simulink model "ML_UAV_3D_2"  (R2018a)
settings: Solver=ode4  StartTime=0.0  StopTime=130  FixedStep=Ts  MaxStep=2*T  MinStep=T  RelTol=1e-4
values from neighbouring files (symbols this model uses):
  Ac = 0.0331    [init_ML_UAV_3D_2.m]
  Am1_LPF = sysd.denominator{1}    [init_ML_UAV_3D_2.m]
  Am2_LPF = sysd.denominator{1}    [init_ML_UAV_3D_2.m]
  Am_coup_LPF = sysd.denominator{1}    [init_ML_UAV_3D_2.m]
  Amp_sf = 3    [init_ML_UAV_3D_2.m]
  Amp_sf_rp = 0.05*uav.m*g    [init_ML_UAV_3D_2.m]
  Bm1_LPF = sysd.numerator{1}    [init_ML_UAV_3D_2.m]
  Bm2_LPF = sysd.numerator{1}    [init_ML_UAV_3D_2.m]
  Bm_coup_LPF = sysd.numerator{1}    [init_ML_UAV_3D_2.m]
  C_S = [5;5;9]*10^-3    [init_ML_UAV_3D_2.m]
  Cd_u = 0.2    [init_ML_UAV_3D_2.m]
  dc_M_p = 6.7    [init_ML_UAV_3D_2.m]
  eps_V = 0.5    [init_ML_UAV_3D_2.m]
  g = 9.81    [init_ML_UAV_3D_2.m]
  gamma_d_p = (2*0.3/0.03*2*0.2*12/4)/10    (= 2.4)    [init_ML_UAV_3D_2.m]
  k3 = 24    [init_ML_UAV_3D_2.m]
  k4 = 0.8    [init_ML_UAV_3D_2.m]
  min_sf = 5    [init_ML_UAV_3D_2.m]
  min_sf_rp = 0.35*uav.m*g    [init_ML_UAV_3D_2.m]
  OMEGA_FILTER_OUTER = 40    [estimation.m]
  T_init = 10    [init_ML_UAV_3D_2.m]
  Tc = 1/500    (= 0.002)    [estimation.m]
  Tg = 1/ 20    (= 0.05)    [estimation.m]
  Tn = 1/500    (= 0.002)    [estimation.m]
  Ts = 1/500    (= 0.002)    [estimation.m]    (also in init_ML_UAV_3D_2.m)
  Tsc = 1/100    (= 0.01)    [estimation.m]
  Tz = 1/500    (= 0.002)    [estimation.m]
  X_GPS_offset = [0.01 0.005]    [estimation.m]
undefined symbols (not defined in the file or in its folder): Am_HPF, Am_LPF, Am_LPF2, an1, an1_v, an2, an3, Bm_HPF, Bm_LPF, Bm_LPF2, bn1, bn1_v, bn2, bn3, buoy, cable, controller, current, D_b, DiscIntNeverNeededParam, F, filters, J_u, K, kd_t, kp_t, L, Light, magnitude, MIL, Phi0, Psi0, R_b, T, Theta0, theta_q_ini, tolerences, torque_corr, uav, Vol_b, water, wave, X0_u
libraries: simulink x48, simulink_extras x10, UAV_Control x4, dspmtrx3 x2, aerolibwind2 x2
(part 3 of 6)

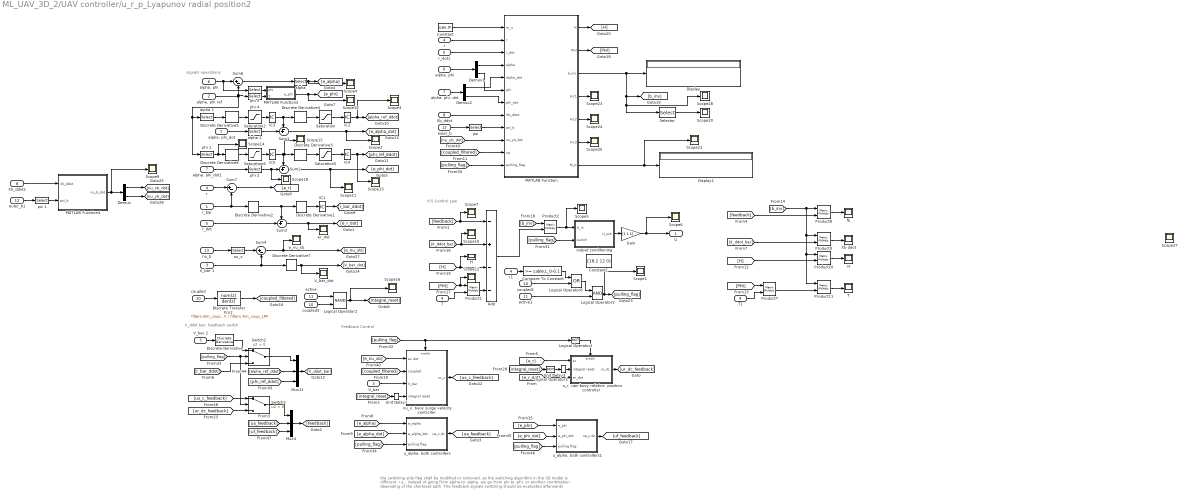
== system ML_UAV_3D_2/UAV controller/u_r_p_Lyapunov radial position2 ==
  note: the switching side flag shall be modified or removed, as the switching algorithm in the 3D model is different.
      | i.e., instead of going from alpha to -alpha, we go from phi to -phi, or another combination depending of the shorteset path.
      |
      | The feedback signals switching should be evaluated afterwards
  note: Feedback Control
  note: ICS Control Law
  note: X_ddot bar, feedbach switch
  note: signals operations
  "r_bar " : Inport
  "alpha, phi ref" : Inport  Port=2
  "V_bar " : Inport  Port=3
  r : Inport  Port=4
  r_dot : Inport  Port=5
  "alpha, phi" : Inport  Port=6
  "alpha, phi, dot" : Inport  Port=7
  Xb_ddot : Inport  Port=8
  T : Inport  Port=9
  coupled : Inport  Port=10
  active : Inport  Port=11
  euler_b : Inport  Port=12
  nu_b : Inport  Port=13
  " H " : Scope
  " H  " : Scope
  " T  " : Scope
  " alpha " : Selector  InputPortWidth=2  IndexOptions=Index vector (dialog)  Indices=1  OutputSizes=1
  " alpha 1" : Selector  InputPortWidth=2  IndexOptions=Index vector (dialog)  Indices=1  OutputSizes=1
  " alpha 2" : Selector  InputPortWidth=2  IndexOptions=Index vector (dialog)  Indices=1  OutputSizes=1
  " fb " : Scope
   phi {1..2,4..5} (4 alike) : Selector  InputPortWidth=2  IndexOptions=Index vector (dialog)  Indices=2  OutputSizes=1
  Add : Sum  Inputs=-+--
  Compare To Constant : simulink/Logic and Bit Operations/Compare To Constant  relop=>=  const=cable.L_0-0.1  OutDataTypeStr=boolean
  Constant : Constant  Value=uav.m
  Constant1 : Constant  Value=[18.2 12 0]
  Demux : Demux  Outputs=2
  Demux1 : Demux  Outputs=2
  Demux2 : Demux  Outputs=2
  Discrete Transfer Fcn2 : DiscreteTransferFcn  Numerator=filters.Bm_coup_LPF  Denominator=filters.Am_coup_LPF
  Discrete Derivative : simulink/Discrete/Discrete Derivative  gainval=1.0  ICPrevScaledInput=0.0  OutMin=[]  OutMax=[]  OutDataType=fixdt(1, 16)  OutScaling=2^-10  DoSatur=off
  Discrete Derivative1 : simulink/Discrete/Discrete Derivative  gainval=1.0  ICPrevScaledInput=uav.r_0/Ts  OutMin=[]  OutMax=[]  OutDataType=fixdt(1, 16)  OutScaling=2^-10  DoSatur=off
  Discrete Derivative2 : simulink/Discrete/Discrete Derivative  gainval=1.0  ICPrevScaledInput=uav.r_0/Ts  OutMin=[]  OutMax=[]  OutDataType=fixdt(1, 16)  OutScaling=2^-10  DoSatur=off
  Discrete Derivative3 : simulink/Discrete/Discrete Derivative  gainval=1.0  ICPrevScaledInput=alpha_bar  OutMin=[]  OutMax=[]  OutDataType=fixdt(1, 16)  OutScaling=2^-10  DoSatur=off
  Discrete Derivative4 : simulink/Discrete/Discrete Derivative  gainval=1.0  ICPrevScaledInput=alpha_bar  OutMin=[]  OutMax=[]  OutDataType=fixdt(1, 16)  OutScaling=2^-10  DoSatur=off
  Discrete Derivative5 : simulink/Discrete/Discrete Derivative  gainval=1.0  ICPrevScaledInput=uav.alpha_bar_0/Ts  OutMin=[]  OutMax=[]  OutDataType=fixdt(1, 16)  OutScaling=2^-10  DoSatur=off
  Discrete Derivative6 : simulink/Discrete/Discrete Derivative  gainval=1.0  ICPrevScaledInput=uav.phi_0/Ts  OutMin=[]  OutMax=[]  OutDataType=fixdt(1, 16)  OutScaling=2^-10  DoSatur=off
  Discrete Derivative7 : simulink/Discrete/Discrete Derivative  gainval=1.0  ICPrevScaledInput=uav.r_0/Ts  OutMin=[]  OutMax=[]  OutDataType=fixdt(1, 16)  OutScaling=2^-10  DoSatur=off
  Display : Display
  Display1 : Display
  Gain : Gain  Gain=[1 1 1]
  IC{1..5} (5 alike) : InitialCondition  Value=0
  Logical Operator1 : Logic  Operator=NOT  AllPortsSameDT=off  OutDataTypeStr=boolean
  Logical Operator2 : Logic  Operator=NAND  AllPortsSameDT=off  OutDataTypeStr=boolean
  Logical Operator3 : Logic  Operator=NOT  AllPortsSameDT=off  OutDataTypeStr=boolean
  Logical Operator5 : Logic  AllPortsSameDT=off  OutDataTypeStr=boolean
  Logical Operator6 : Logic  Operator=OR  AllPortsSameDT=off  OutDataTypeStr=boolean
  MATLAB Function : MATLAB Function  TreatAsAtomicUnit=on
  MATLAB Function2 : MATLAB Function  TreatAsAtomicUnit=on
  MATLAB Function4 : MATLAB Function  TreatAsAtomicUnit=on
  Mux11 : Mux  Inputs=3
  Mux4 : Mux  Inputs=3
  Product{1..2,7..11} (7 alike) : Product  Inputs=**  Multiplication=Matrix(*)
  Saturation : Saturate  UpperLimit=2  LowerLimit=-2
  Saturation2 : Saturate  UpperLimit=1  LowerLimit=-1
  Saturation5 : Saturate  UpperLimit=2  LowerLimit=-2
  Saturation6 : Saturate  UpperLimit=1  LowerLimit=-1
  Scope{1..7,9..16,18..21,23..25,27..28} (24 alike) : Scope
  Selector : Selector  NumberOfDimensions=2  InputPortWidth=3  IndexOptions=Index vector (dialog),Index vector (dialog)  Indices=[2 3],[3 3]  OutputSizes=1,1
  Sum1 : Sum  Inputs=-+|
  Sum2 : Sum  Inputs=-+|
  Sum3 : Sum  Inputs=-+|
  Sum4 : Sum  Inputs=|+-
  Sum6 : Sum  Inputs=|+-
  Sum7 : Sum  Inputs=|+-
  Switch2 : Switch  Criteria=u2 > Threshold
  Switch3 : Switch  Criteria=u2 > Threshold
  T1 : InportShadow  Port=9
  Unit Delay1 : UnitDelay  SampleTime=-1
  Unit Delay3 : UnitDelay  SampleTime=-1
  V_bar 1 : InportShadow  Port=3
  V_bar 2 : InportShadow  Port=3
  V_bar_dot : Scope
  "Xb ddot " : Scope
  Xb_ddot1 : InportShadow  Port=8
  active1 : InportShadow  Port=11
  "alpha, phi " : InportShadow  Port=6
  "alpha, phi_dot" : InportShadow  Port=7
  "alpha, phi_dot1" : InportShadow  Port=7
  coupled1 : InportShadow  Port=10
  coupled3 : InportShadow  Port=10
  e_nu_xb : Scope
  er_dot : Scope
  euler_b1 : InportShadow  Port=12
  nu_x : Selector  InputPortWidth=2  IndexOptions=Index vector (dialog)  Indices=1  OutputSizes=1
  "nu_x, buoy surge velocity controller" : Subsystem
  output conditioning : Subsystem
  "psi " : Selector  InputPortWidth=3  IndexOptions=Index vector (dialog)  Indices=3  OutputSizes=1
  psi 1 : Selector  InputPortWidth=3  IndexOptions=Index vector (dialog)  Indices=3  OutputSizes=1
  "r  " : InportShadow  Port=4
  r1 : InportShadow  Port=4
  r_dot1 : InportShadow  Port=5
  "u_alpha, both controllers" : Subsystem
  "u_alpha, both controllers1" : Subsystem
  "u_r, uav-buoy relative  position controller" : Subsystem
  U : Outport
  wires:
  r_dot/1 -> Sum3/2
  [feedback] -> Add/1, Scope7/1
  r_dot1/1 -> MATLAB Function/3(r_dot)
  Discrete Derivative2/1 -> Discrete Derivative1/1, Sum3/1
  Discrete Derivative4/1 -> Saturation/1
  Saturation2/1 -> IC3/1
  " alpha 1"/1 -> Discrete Derivative5/1
  Discrete Derivative5/1 -> Saturation2/1
  IC3/1 -> Discrete Derivative4/1, Sum1/1
  Saturation/1 -> IC2/1
  [coupled_filtered] -> MATLAB Function/11(cp)
  coupled3/1 -> Logical Operator2/2
  coupled/1 -> Discrete Transfer Fcn2/1
  active/1 -> Logical Operator2/1
  "alpha, phi "/1 -> " phi 5"/1, Sum6/1
  "alpha, phi ref"/1 -> " phi 1"/1, " alpha 1"/1, " phi 4"/1, Sum6/2
  Sum6/1 -> " alpha "/1
  " alpha "/1 -> Scope4/1, [e_alpha]
  MATLAB Function2/1(e_phi) -> Scope19/1, [e_phi]
  "r  "/1 -> Sum7/1
  "r_bar "/1 -> Discrete Derivative2/1, Sum7/2
  Sum7/1 -> [e_r]
  Discrete Derivative1/1 -> IC1/1
  IC2/1 -> Scope3/1, [alpha_ref_ddot]
  " phi 1"/1 -> Scope14/1, Discrete Derivative6/1
  Discrete Derivative3/1 -> Saturation5/1
  Discrete Derivative6/1 -> Saturation6/1
  IC4/1 -> Scope13/1, [phi_ref_ddot]
  Saturation6/1 -> IC5/1
  Saturation5/1 -> IC4/1
  IC1/1 -> [r_bar_ddot]
  Sum3/1 -> er_dot/1, [e_r_dot]
  "alpha, phi_dot"/1 -> " alpha 2"/1
  Sum1/1 -> Scope2/1, [e_alpha_dot]
  " alpha 2"/1 -> Sum1/2
  "alpha, phi_dot1"/1 -> " phi 2"/1
  " phi 2"/1 -> Scope18/1, Sum2/2
  IC5/1 -> Scope15/1, Discrete Derivative3/1, Sum2/1
  Sum2/1 -> [e_phi_dot], Scope11/1
  Discrete Transfer Fcn2/1 -> [coupled_filtered]
  "alpha, phi"/1 -> Demux1/1
  Demux1/1 -> MATLAB Function/4(alpha)
  Demux1/2 -> MATLAB Function/6(phi)
  Demux2/1 -> MATLAB Function/5(alpha_dot)
  Demux2/2 -> MATLAB Function/7(phi_dot)
  "alpha, phi, dot"/1 -> Demux2/1
  Xb_ddot/1 -> MATLAB Function/8(Xb_ddot)
  [pulling_flag] -> MATLAB Function/12(pulling_flag)
  r/1 -> MATLAB Function/2(r)
  [phi_ref_ddot] -> Mux11/3
  [alpha_ref_ddot] -> Mux11/2
  [pulling_flag] -> Switch2/2, Switch3/2
  Discrete Derivative/1 -> Switch2/1
  [r_bar_ddot] -> Switch2/3
  Switch2/1 -> Mux11/1
  [X_ddot_bar] -> Add/2, Scope10/1
  MATLAB Function/2(PHI) -> [PHI]
  [PHI] -> Scope12/1, Product1/1
  T/1 -> Product1/2
  Product1/1 -> Add/4
  [b_inv] -> Product2/1
  MATLAB Function/1(H) -> [H]
  Constant/1 -> MATLAB Function/1(m_u)
  [ur_dc_feedback] -> Switch3/3
  [ua_feedback] -> Mux4/2
  Logical Operator2/1 -> Scope16/1, [integral_reset]
  [e_nu_xb] -> "nu_x, buoy surge velocity controller"/1(ex dot)
  [coupled_filtered] -> "nu_x, buoy surge velocity controller"/2(coupled)
  "V_bar "/1 -> "nu_x, buoy surge velocity controller"/3(V_bar)
  [integral_reset] -> Unit Delay1/1
  "nu_x, buoy surge velocity controller"/1(ux_c) -> [ux_c_feedback]
  [e_r] -> "u_r, uav-buoy relative  position controller"/1(er)
  [integral_reset] -> Logical Operator3/1
  [e_r_dot] -> "u_r, uav-buoy relative  position controller"/3(er_dot)
  "u_r, uav-buoy relative  position controller"/1(ur_dc) -> [ur_dc_feedback]
  Logical Operator3/1 -> Unit Delay3/1
  [e_alpha] -> "u_alpha, both controllers"/1(e_alpha)
  [e_alpha_dot] -> "u_alpha, both controllers"/2(e_alpha_dot)
  "u_alpha, both controllers"/1(ua_c,dc) -> [ua_feedback]
  [ux_c_feedback] -> Switch3/1
  Switch3/1 -> Mux4/1
  [pulling_flag] -> output conditioning/2(switch)
  Unit Delay1/1 -> "nu_x, buoy surge velocity controller"/4(integral reset)
  Unit Delay3/1 -> "u_r, uav-buoy relative  position controller"/2(integral reset)
  Logical Operator1/1 -> "u_r, uav-buoy relative  position controller"/Enable
  r1/1 -> Compare To Constant/1
  active1/1 -> Logical Operator5/2
  Logical Operator6/1 -> Logical Operator5/1
  coupled1/1 -> Logical Operator6/2
  Compare To Constant/1 -> Logical Operator6/1
  Logical Operator5/1 -> Scope1/1, [pulling_flag]
  output conditioning/1(U_out) -> Gain/1
  Gain/1 -> Scope6/1, U/1
  Add/1 -> Product2/2
  [pulling_flag] -> "u_alpha, both controllers"/3(pulling flag)
  Selector/1 -> Scope20/1
  MATLAB Function/4(Hc1) -> Scope23/1
  MATLAB Function/5(Hc2) -> Scope24/1
  MATLAB Function/6(Hc3) -> Scope25/1
  MATLAB Function/3(b_inv) -> Display/1, [b_inv], Selector/1, Scope28/1
  " phi 4"/1 -> MATLAB Function2/2(phi_cmd)
  " phi 5"/1 -> MATLAB Function2/1(phi)
  [H] -> Add/3, " H  "/1
  Product2/1 -> output conditioning/1(U_in), Scope5/1
  euler_b/1 -> "psi "/1
  "psi "/1 -> MATLAB Function/9(psi_b)
  Sum4/1 -> e_nu_xb/1, [e_nu_xb]
  nu_b/1 -> nu_x/1
  [nu_yb_dot] -> MATLAB Function/10(nu_yb_dot)
  V_bar 2/1 -> Discrete Derivative/1
  [pulling_flag] -> "u_alpha, both controllers1"/3(pulling flag)
  [e_phi_dot] -> "u_alpha, both controllers1"/2(e_phi_dot)
  [e_phi] -> "u_alpha, both controllers1"/1(e_phi)
  "u_alpha, both controllers1"/1(ua_c,dc) -> [uf_feedback]
  [uf_feedback] -> Mux4/3
  Xb_ddot1/1 -> MATLAB Function4/1(Xb_ddot)
  euler_b1/1 -> psi 1/1
  psi 1/1 -> MATLAB Function4/2(psi_b)
  MATLAB Function4/1(nu_b_dot) -> Scope9/1, Demux/1
  Demux/1 -> [nu_xb_dot]
  Demux/2 -> [nu_yb_dot]
  MATLAB Function/7(M_p) -> Display1/1, Scope21/1
  [pulling_flag] -> "nu_x, buoy surge velocity controller"/Enable, Logical Operator1/1
  Mux11/1 -> [X_ddot_bar]
  Mux4/1 -> [feedback]
  [PHI] -> Product7/1
  T1/1 -> Product7/2
  Product8/1 -> " fb "/1
  [feedback] -> Product8/2
  Product7/1 -> Product11/2
  [H] -> Product10/2
  [X_ddot_bar] -> Product9/2
  [b_inv] -> Product11/1, Product10/1, Product9/1, Product8/1
  Product9/1 -> "Xb ddot "/1
  Product10/1 -> " H "/1
  Product11/1 -> " T  "/1
  nu_x/1 -> Sum4/1
  V_bar 1/1 -> Discrete Derivative7/1, Sum4/2
  Discrete Derivative7/1 -> V_bar_dot/1, [V_bar_dot]

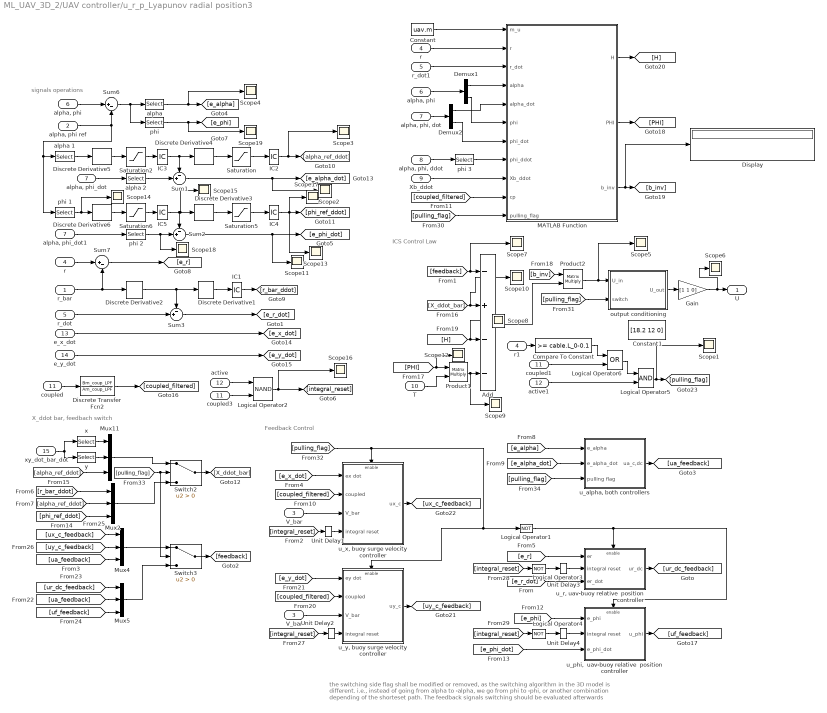
== system ML_UAV_3D_2/UAV controller/u_r_p_Lyapunov radial position3 ==
  note: the switching side flag shall be modified or removed, as the switching algorithm in the 3D model is different.
      | i.e., instead of going from alpha to -alpha, we go from phi to -phi, or another combination depending of the shorteset path.
      |
      | The feedback signals switching should be evaluated afterwards
  note: Feedback Control
  note: ICS Control Law
  note: X_ddot bar, feedbach switch
  note: signals operations
  "r_bar " : Inport
  "alpha, phi ref" : Inport  Port=2
  "V_bar " : Inport  Port=3
  r : Inport  Port=4
  r_dot : Inport  Port=5
  "alpha, phi" : Inport  Port=6
  "alpha, phi, dot" : Inport  Port=7
  "alpha, phi, ddot" : Inport  Port=8
  Xb_ddot : Inport  Port=9
  T : Inport  Port=10
  coupled : Inport  Port=11
  active : Inport  Port=12
  e_x_dot : Inport  Port=13
  e_y_dot : Inport  Port=14
  xy_dot_bar_dot : Inport  Port=15
  " alpha " : Selector  InputPortWidth=2  IndexOptions=Index vector (dialog)  Indices=1  OutputSizes=1
  " alpha 1" : Selector  InputPortWidth=2  IndexOptions=Index vector (dialog)  Indices=1  OutputSizes=1
  " alpha 2" : Selector  InputPortWidth=2  IndexOptions=Index vector (dialog)  Indices=1  OutputSizes=1
   phi {,1..3} (4 alike) : Selector  InputPortWidth=2  IndexOptions=Index vector (dialog)  Indices=2  OutputSizes=1
  " x " : Selector  InputPortWidth=2  IndexOptions=Index vector (dialog)  Indices=1  OutputSizes=1
  " y " : Selector  InputPortWidth=2  IndexOptions=Index vector (dialog)  Indices=2  OutputSizes=1
  Add : Sum  Inputs=-+--
  Compare To Constant : simulink/Logic and Bit Operations/Compare To Constant  relop=>=  const=cable.L_0-0.1  OutDataTypeStr=boolean
  Constant : Constant  Value=uav.m
  Constant1 : Constant  Value=[18.2 12 0]
  Demux1 : Demux  Outputs=2
  Demux2 : Demux  Outputs=2
  Discrete Transfer Fcn2 : DiscreteTransferFcn  Numerator=Bm_coup_LPF  Denominator=Am_coup_LPF
  Discrete Derivative1 : simulink/Discrete/Discrete Derivative  gainval=1.0  ICPrevScaledInput=uav.r_0/Ts  OutMin=[]  OutMax=[]  OutDataType=fixdt(1, 16)  OutScaling=2^-10  DoSatur=off
  Discrete Derivative2 : simulink/Discrete/Discrete Derivative  gainval=1.0  ICPrevScaledInput=uav.r_0/Ts  OutMin=[]  OutMax=[]  OutDataType=fixdt(1, 16)  OutScaling=2^-10  DoSatur=off
  Discrete Derivative3 : simulink/Discrete/Discrete Derivative  gainval=1.0  ICPrevScaledInput=alpha_bar  OutMin=[]  OutMax=[]  OutDataType=fixdt(1, 16)  OutScaling=2^-10  DoSatur=off
  Discrete Derivative4 : simulink/Discrete/Discrete Derivative  gainval=1.0  ICPrevScaledInput=alpha_bar  OutMin=[]  OutMax=[]  OutDataType=fixdt(1, 16)  OutScaling=2^-10  DoSatur=off
  Discrete Derivative5 : simulink/Discrete/Discrete Derivative  gainval=1.0  ICPrevScaledInput=uav.alpha_bar_0/Ts  OutMin=[]  OutMax=[]  OutDataType=fixdt(1, 16)  OutScaling=2^-10  DoSatur=off
  Discrete Derivative6 : simulink/Discrete/Discrete Derivative  gainval=1.0  ICPrevScaledInput=uav.phi_0/Ts  OutMin=[]  OutMax=[]  OutDataType=fixdt(1, 16)  OutScaling=2^-10  DoSatur=off
  Display : Display
  Gain : Gain  Gain=[1 1 0]
  IC{1..5} (5 alike) : InitialCondition  Value=0
  Logical Operator1 : Logic  Operator=NOT  AllPortsSameDT=off  OutDataTypeStr=boolean
  Logical Operator2 : Logic  Operator=NAND  AllPortsSameDT=off  OutDataTypeStr=boolean
  Logical Operator3 : Logic  Operator=NOT  AllPortsSameDT=off  OutDataTypeStr=boolean
  Logical Operator4 : Logic  Operator=NOT  AllPortsSameDT=off  OutDataTypeStr=boolean
  Logical Operator5 : Logic  AllPortsSameDT=off  OutDataTypeStr=boolean
  Logical Operator6 : Logic  Operator=OR  AllPortsSameDT=off  OutDataTypeStr=boolean
  MATLAB Function : MATLAB Function  TreatAsAtomicUnit=on
  Mux{2,4..5,11} (4 alike) : Mux  Inputs=3
  Product1 : Product  Inputs=**  Multiplication=Matrix(*)
  Product2 : Product  Inputs=**  Multiplication=Matrix(*)
  Saturation : Saturate  UpperLimit=2  LowerLimit=-2
  Saturation2 : Saturate  UpperLimit=1  LowerLimit=-1
  Saturation5 : Saturate  UpperLimit=2  LowerLimit=-2
  Saturation6 : Saturate  UpperLimit=1  LowerLimit=-1
  Scope{1..19} (19 alike) : Scope
  Sum1 : Sum  Inputs=-+|
  Sum2 : Sum  Inputs=-+|
  Sum3 : Sum  Inputs=-+|
  Sum6 : Sum  Inputs=|+-
  Sum7 : Sum  Inputs=|+-
  Switch2 : Switch  Criteria=u2 > Threshold
  Switch3 : Switch  Criteria=u2 > Threshold
  Unit Delay{1..4} (4 alike) : UnitDelay  SampleTime=-1
  V_bar : InportShadow  Port=3
  active1 : InportShadow  Port=12
  "alpha, phi " : InportShadow  Port=6
  "alpha, phi_dot" : InportShadow  Port=7
  "alpha, phi_dot1" : InportShadow  Port=7
  coupled1 : InportShadow  Port=11
  coupled3 : InportShadow  Port=11
  output conditioning : Subsystem
  "r  " : InportShadow  Port=4
  r1 : InportShadow  Port=4
  r_dot1 : InportShadow  Port=5
  "u_alpha, both controllers" : Subsystem
  "u_phi,  uav-buoy relative  position controller" : Subsystem
  "u_r, uav-buoy relative  position controller" : Subsystem
  "u_x, buoy surge velocity controller" : Subsystem
  "u_y, buoy surge velocity controller" : Subsystem
  U : Outport
  wires:
  r_dot/1 -> Sum3/2
  [feedback] -> Scope7/1, Add/1
  [r_bar_ddot] -> Mux2/1
  r_dot1/1 -> MATLAB Function/3(r_dot)
  Discrete Derivative2/1 -> Discrete Derivative1/1, Sum3/1
  [ux_c_feedback] -> Mux4/1
  Discrete Derivative4/1 -> Saturation/1
  Saturation2/1 -> IC3/1
  " alpha 1"/1 -> Discrete Derivative5/1
  Discrete Derivative5/1 -> Saturation2/1
  IC3/1 -> Discrete Derivative4/1, Sum1/1
  Saturation/1 -> IC2/1
  [alpha_ref_ddot] -> Mux2/2
  [coupled_filtered] -> MATLAB Function/10(cp)
  coupled3/1 -> Logical Operator2/2
  coupled/1 -> Discrete Transfer Fcn2/1
  active/1 -> Logical Operator2/1
  "alpha, phi "/1 -> Sum6/1
  "alpha, phi ref"/1 -> " phi 1"/1, " alpha 1"/1, Sum6/2
  Sum6/1 -> " phi "/1, " alpha "/1
  " alpha "/1 -> Scope4/1, [e_alpha]
  " phi "/1 -> Scope19/1, [e_phi]
  "r  "/1 -> Sum7/1
  "r_bar "/1 -> Discrete Derivative2/1, Sum7/2
  Sum7/1 -> [e_r]
  Discrete Derivative1/1 -> IC1/1
  IC2/1 -> Scope3/1, [alpha_ref_ddot]
  " phi 1"/1 -> Scope14/1, Discrete Derivative6/1
  Discrete Derivative3/1 -> Saturation5/1
  Discrete Derivative6/1 -> Saturation6/1
  IC4/1 -> Scope17/1, Scope13/1, [phi_ref_ddot]
  Saturation6/1 -> IC5/1
  Saturation5/1 -> IC4/1
  IC1/1 -> [r_bar_ddot]
  Sum3/1 -> [e_r_dot]
  "alpha, phi_dot"/1 -> " alpha 2"/1
  Sum1/1 -> Scope2/1, [e_alpha_dot]
  " alpha 2"/1 -> Sum1/2
  "alpha, phi_dot1"/1 -> " phi 2"/1
  " phi 2"/1 -> Scope18/1, Sum2/2
  IC5/1 -> Scope15/1, Discrete Derivative3/1, Sum2/1
  Sum2/1 -> Scope11/1, [e_phi_dot]
  Discrete Transfer Fcn2/1 -> [coupled_filtered]
  [phi_ref_ddot] -> Mux2/3
  "alpha, phi"/1 -> Demux1/1
  Demux1/1 -> MATLAB Function/4(alpha)
  Demux1/2 -> MATLAB Function/6(phi)
  Demux2/1 -> MATLAB Function/5(alpha_dot)
  Demux2/2 -> MATLAB Function/7(phi_dot)
  "alpha, phi, dot"/1 -> Demux2/1
  Xb_ddot/1 -> MATLAB Function/9(Xb_ddot)
  "alpha, phi, ddot"/1 -> " phi 3"/1
  " phi 3"/1 -> MATLAB Function/8(phi_ddot)
  [pulling_flag] -> MATLAB Function/11(pulling_flag)
  r/1 -> MATLAB Function/2(r)
  [alpha_ref_ddot] -> Mux11/3
  " x "/1 -> Mux11/1
  xy_dot_bar_dot/1 -> " y "/1, " x "/1
  " y "/1 -> Mux11/2
  [pulling_flag] -> Switch2/2, Switch3/2
  Mux11/1 -> Switch2/1
  Mux2/1 -> Switch2/3
  Switch2/1 -> [X_ddot_bar]
  [X_ddot_bar] -> Scope10/1, Add/2
  MATLAB Function/2(PHI) -> [PHI]
  [PHI] -> Scope12/1, Product1/1
  T/1 -> Product1/2
  Product1/1 -> Scope9/1, Add/4
  MATLAB Function/3(b_inv) -> Display/1, [b_inv]
  [b_inv] -> Product2/1
  MATLAB Function/1(H) -> [H]
  [H] -> Scope8/1, Add/3
  Constant/1 -> MATLAB Function/1(m_u)
  [ur_dc_feedback] -> Mux5/1
  [ua_feedback] -> Mux5/2
  [uf_feedback] -> Mux5/3
  [ua_feedback] -> Mux4/3
  [uy_c_feedback] -> Mux4/2
  Logical Operator2/1 -> Scope16/1, [integral_reset]
  [e_x_dot] -> "u_x, buoy surge velocity controller"/1(ex dot)
  [coupled_filtered] -> "u_x, buoy surge velocity controller"/2(coupled)
  "V_bar "/1 -> "u_x, buoy surge velocity controller"/3(V_bar)
  [integral_reset] -> Unit Delay1/1
  "u_x, buoy surge velocity controller"/1(ux_c) -> [ux_c_feedback]
  [e_y_dot] -> "u_y, buoy surge velocity controller"/1(ey dot)
  [coupled_filtered] -> "u_y, buoy surge velocity controller"/2(coupled)
  V_bar/1 -> "u_y, buoy surge velocity controller"/3(V_bar)
  [integral_reset] -> Unit Delay2/1
  "u_y, buoy surge velocity controller"/1(uy_c) -> [uy_c_feedback]
  [e_phi] -> "u_phi,  uav-buoy relative  position controller"/1(e_phi)
  [e_phi_dot] -> "u_phi,  uav-buoy relative  position controller"/3(e_phi_dot)
  "u_phi,  uav-buoy relative  position controller"/1(u_phi) -> [uf_feedback]
  [e_r] -> "u_r, uav-buoy relative  position controller"/1(er)
  [integral_reset] -> Logical Operator3/1
  [e_r_dot] -> "u_r, uav-buoy relative  position controller"/3(er_dot)
  "u_r, uav-buoy relative  position controller"/1(ur_dc) -> [ur_dc_feedback]
  Logical Operator3/1 -> Unit Delay3/1
  [e_alpha] -> "u_alpha, both controllers"/1(e_alpha)
  [e_alpha_dot] -> "u_alpha, both controllers"/2(e_alpha_dot)
  "u_alpha, both controllers"/1(ua_c,dc) -> [ua_feedback]
  Mux4/1 -> Switch3/1
  Mux5/1 -> Switch3/3
  Switch3/1 -> [feedback]
  [pulling_flag] -> output conditioning/2(switch)
  [pulling_flag] -> Logical Operator1/1, "u_y, buoy surge velocity controller"/Enable, "u_x, buoy surge velocity controller"/Enable
  Unit Delay1/1 -> "u_x, buoy surge velocity controller"/4(integral reset)
  Unit Delay2/1 -> "u_y, buoy surge velocity controller"/4(integral reset)
  Unit Delay3/1 -> "u_r, uav-buoy relative  position controller"/2(integral reset)
  Logical Operator4/1 -> Unit Delay4/1
  [integral_reset] -> Logical Operator4/1
  Unit Delay4/1 -> "u_phi,  uav-buoy relative  position controller"/2(integral reset)
  Logical Operator1/1 -> "u_phi,  uav-buoy relative  position controller"/Enable, "u_r, uav-buoy relative  position controller"/Enable
  r1/1 -> Compare To Constant/1
  active1/1 -> Logical Operator5/2
  Logical Operator6/1 -> Logical Operator5/1
  coupled1/1 -> Logical Operator6/2
  Compare To Constant/1 -> Logical Operator6/1
  Logical Operator5/1 -> Scope1/1, [pulling_flag]
  e_x_dot/1 -> [e_x_dot]
  e_y_dot/1 -> [e_y_dot]
  Product2/1 -> Scope5/1, output conditioning/1(U_in)
  output conditioning/1(U_out) -> Gain/1
  Gain/1 -> U/1, Scope6/1
  Add/1 -> Product2/2
  [pulling_flag] -> "u_alpha, both controllers"/3(pulling flag)

== system ML_UAV_3D_2/Wind model/magnitude ==
  In1 : Inport
  Math Function2 : Math  Operator=magnitude^2  SaturateOnIntegerOverflow=on
  Sqrt : Sqrt  SaturateOnIntegerOverflow=on
  Sum of Elements1 : Sum  Inputs=+
  Out1 : Outport
  wires:
  Sum of Elements1/1 -> Sqrt/1
  Math Function2/1 -> Sum of Elements1/1
  Sqrt/1 -> Out1/1
  In1/1 -> Math Function2/1

== system ML_UAV_3D_2/Quadrotor+buoy/6-DOF equations of motion Earth frame/C_1-5 ==
  "alpha, phi " : Inport
  "alpha_dot, phi_dot" : Inport  Port=2
  coupled : Inport  Port=3
  Add : Sum
  Add1 : Sum
  Constant1 : Constant  Value=m_u*L
  Demux : Demux  Outputs=2
  Gain1 : Gain  Gain=L
  Gain2 : Gain  Gain=-2
  Ground : Ground
  Product{1,3..10} (9 alike) : Product
  Product2 : Product  Inputs=3
  Signal Specification{4..8} (5 alike) : SignalSpecification  Dimensions=5
  Vector Concatenate : Concatenate
  Vector Concatenate5 : Concatenate  NumInputs=5  Mode=Multidimensional array  ConcatenateDimension=2
  alpha_dot : Concatenate  NumInputs=5
  c_a*c_p : Fcn  Expr=-u(3)*u(4)
  c_a*s_p : Fcn  Expr=-u(3)*u(2)
  phi_dot : Concatenate  NumInputs=5
  s_a : Fcn  Expr=-u(1)
  s_a*c_a : Fcn  Expr=u(1)*u(3)
  s_a*c_p : Fcn  Expr=-2*u(1)*u(4)
  s_a*s_p : Fcn  Expr=2*u(1)*u(2)
  s_alpha s_phi c_alpha c_phi : Trigonometry  Operator=sincos
  x_dot : Concatenate  NumInputs=5
  y_dot : Concatenate  NumInputs=5
  z_dot : Concatenate  NumInputs=5
  C_123 : Outport
  wires:
  coupled/1 -> Product2/1
  Constant1/1 -> Product2/2
  Vector Concatenate/1 -> s_a*c_a/1, s_a/1, s_a*c_p/1, c_a*s_p/1, c_a*c_p/1, s_a*s_p/1
  "alpha, phi "/1 -> s_alpha s_phi c_alpha c_phi/1
  s_alpha s_phi c_alpha c_phi/1 -> Vector Concatenate/1
  s_alpha s_phi c_alpha c_phi/2 -> Vector Concatenate/2
  z_dot/1 -> Signal Specification6/1
  Signal Specification7/1 -> Vector Concatenate5/4
  Signal Specification8/1 -> Vector Concatenate5/5
  phi_dot/1 -> Signal Specification8/1
  y_dot/1 -> Signal Specification5/1
  Signal Specification5/1 -> Vector Concatenate5/2
  Signal Specification4/1 -> Vector Concatenate5/1
  x_dot/1 -> Signal Specification4/1
  alpha_dot/1 -> Signal Specification7/1
  Signal Specification6/1 -> Vector Concatenate5/3
  Ground/1 -> x_dot/1, x_dot/2, x_dot/3, x_dot/4, x_dot/5, y_dot/1, y_dot/2, y_dot/3, y_dot/4, y_dot/5, z_dot/1, z_dot/2, z_dot/3, z_dot/4, z_dot/5, alpha_dot/4, phi_dot/3, phi_dot/5  "44"
  Product2/1 -> C_123/1
  Vector Concatenate5/1 -> Product2/3
  s_a*c_a/1 -> Gain1/1
  "alpha_dot, phi_dot"/1 -> Demux/1
  Demux/2 -> Product5/2, Product7/2, Product10/2, Product3/1, Product1/2, Product9/2  "phi_dot"
  Gain1/1 -> Gain2/1, Product3/2
  Product4/1 -> Add/1
  c_a*c_p/1 -> Product9/1, Product4/1
  Demux/1 -> Product8/2, Product4/2, Product6/2  "alpha_dot"
  s_a*s_p/1 -> Product5/1
  Product5/1 -> Add/2
  Add/1 -> alpha_dot/1  "14"
  Product7/1 -> Add1/2
  Product6/1 -> Add1/1
  Add1/1 -> alpha_dot/2  "24"
  c_a*s_p/1 -> Product10/1, Product6/1
  s_a*c_p/1 -> Product7/1
  s_a/1 -> Product8/1
  Product8/1 -> alpha_dot/3  "34"
  Product3/1 -> phi_dot/4  "45"
  Product1/1 -> alpha_dot/5  "54"
  Product9/1 -> phi_dot/1
  Product10/1 -> phi_dot/2
  Gain2/1 -> Product1/1

== system ML_UAV_3D_2/Quadrotor+buoy/6-DOF equations of motion Earth frame/Coupling state ==
  pos_T : Inport
  re_couple : Inport  Port=2
  Data Type Conversion : DataTypeConversion  OutDataTypeStr=double
  Delay10 : Delay  DelayLength=1  InitialCondition=1
  IC3 : InitialCondition
  IC5 : InitialCondition  Value=coupled_ini
  MATLAB Function : MATLAB Function  TreatAsAtomicUnit=on
  "T, r,xu,xb1" : Scope
  break algebraic loop : Delay  DelayLength=1  InitialCondition=1
  "is coupled " : Scope
  is coupled -1 : Scope
  pos tension : Scope
  positive tension : Scope
  "positive tension with gap " : simulink/Logic and Bit Operations/Compare To Constant  relop=>  const=0-0.01  OutDataTypeStr=boolean
  "re_couple " : Scope
  state detector : Scope
  is coupled : Outport
  wires:
  Delay10/1 -> is coupled -1/1, MATLAB Function/3(coupled)
  IC5/1 -> is coupled/1, Delay10/1
  MATLAB Function/1(is_coupled) -> IC5/1, "is coupled "/1
  break algebraic loop/1 -> pos tension/1, MATLAB Function/1(pos_T)
  re_couple/1 -> MATLAB Function/2(re_couple), "re_couple "/1
  MATLAB Function/2(c) -> state detector/1
  pos_T/1 -> "T, r,xu,xb1"/1, "positive tension with gap "/1
  Data Type Conversion/1 -> positive tension/1, break algebraic loop/1
  IC3/1 -> Data Type Conversion/1
  "positive tension with gap "/1 -> IC3/1

== system ML_UAV_3D_2/Quadrotor+buoy/6-DOF equations of motion Earth frame/D_1-5 ==
  eta_dot_tilde : Inport
  Rb : Inport  Port=2
  Rb_T : Inport  Port=3
  dh : Inport  Port=4
  Constant6 : Constant  Value=[0 0 0 0 0]
  Ground : Ground
  Ground1 : Ground
  Ground2 : Ground
  Scope : Scope
  Scope1 : Scope
  Scope2 : Scope
  Signal Specification{1,3..6} (5 alike) : SignalSpecification  Dimensions=5
  Signal Specification2 : SignalSpecification  Dimensions=[5 5]
  "T, r,xu,xb7" : Scope
  Vector Concatenate4 : Concatenate
  Vector Concatenate5 : Concatenate
  Vector Concatenate6 : Concatenate
  Vector Concatenate7 : Concatenate  NumInputs=5  Mode=Multidimensional array  ConcatenateDimension=2
  Water Daming : Subsystem
  Water Daming (simplified : Subsystem  Commented=on
  x_ddot : Concatenate  NumInputs=5
  y_ddot : Concatenate  NumInputs=5
  z_ddot : Concatenate  NumInputs=5
  D_15 : Outport
  wires:
  Water Daming/4(D22_I) -> Vector Concatenate5/2, y_ddot/2
  Water Daming/1(D11_I) -> x_ddot/1, Vector Concatenate4/2
  eta_dot_tilde/1 -> Water Daming/3(eta_dot_tilde)
  dh/1 -> Water Daming/4(dh)
  Vector Concatenate4/1 -> Scope/1
  Water Daming (simplified/1(D11_I) -> Vector Concatenate4/1
  Vector Concatenate5/1 -> Scope1/1
  Water Daming (simplified/4(D22_I) -> Vector Concatenate5/1
  Vector Concatenate6/1 -> Scope2/1
  Water Daming (simplified/6(D33_I) -> Vector Concatenate6/1
  Signal Specification2/1 -> D_15/1
  Rb/1 -> Water Daming (simplified/1(euler_b), Water Daming/1(Rb)
  z_ddot/1 -> Signal Specification4/1
  Signal Specification5/1 -> Vector Concatenate7/4
  Signal Specification6/1 -> Vector Concatenate7/5
  Constant6/1 -> Signal Specification6/1, Signal Specification5/1
  y_ddot/1 -> Signal Specification3/1
  Signal Specification3/1 -> Vector Concatenate7/2
  Signal Specification1/1 -> Vector Concatenate7/1
  x_ddot/1 -> Signal Specification1/1, "T, r,xu,xb7"/1
  Signal Specification4/1 -> Vector Concatenate7/3
  Vector Concatenate7/1 -> Signal Specification2/1
  Water Daming/2(D12_I) -> y_ddot/1, x_ddot/2
  Water Daming/3(D13_I) -> x_ddot/3, z_ddot/1
  Ground/1 -> x_ddot/5, x_ddot/4
  Ground1/1 -> y_ddot/5, y_ddot/4
  Ground2/1 -> z_ddot/5, z_ddot/4
  Water Daming/5(D23_I) -> z_ddot/2, y_ddot/3
  Water Daming/6(D33_I) -> Vector Concatenate6/2, z_ddot/3
  Rb_T/1 -> Water Daming/2(Rb_T)

== system ML_UAV_3D_2/Quadrotor+buoy/6-DOF equations of motion Earth frame/D_u (vector for simplification) ==
  Vr : Inport
  A.Q.Cd : Product
  Abs : Abs
  Cd x A : Constant  Value=Cd_u*Ac
  rho/2 : Gain  Gain=rho_a/2
  Du : Outport
  wires:
  Vr/1 -> Abs/1
  Cd x A/1 -> A.Q.Cd/2
  rho/2/1 -> A.Q.Cd/1
  Abs/1 -> rho/2/1
  A.Q.Cd/1 -> Du/1

== system ML_UAV_3D_2/Quadrotor+buoy/6-DOF equations of motion Earth frame/FB ==
  Constant1 : Constant  Value=rho_w*g
  F_B : Product
  Out1 : Outport
  wires:
  F_B/1 -> Out1/1
  [Vol_im] -> F_B/1
  Constant1/1 -> F_B/2

== system ML_UAV_3D_2/Quadrotor+buoy/6-DOF equations of motion Earth frame/G1 ==
  Constant3 : Constant  Value=0
  Constant4 : Constant  Value=(m_b)*g
  Vector Concatenate : Concatenate
  G : Outport
  wires:
  Vector Concatenate/1 -> G/1
  Constant3/1 -> Vector Concatenate/1  "u1"
  Constant4/1 -> Vector Concatenate/2  "u2"

== system ML_UAV_3D_2/Quadrotor+buoy/6-DOF equations of motion Earth frame/G1-5 ==
  alpha : Inport
  coupled : Inport  Port=2
  Constant : Constant  Value=m_b
  Constant4 : Constant  Value=m_u
  Constant5 : Constant  Value=g*L
  Gain1 : Gain  Gain=g
  Ground : Ground
  Product : Product
  Product5 : Product  Inputs=3  SaturateOnIntegerOverflow=on  InputSameDT=on  OutDataTypeStr=Inherit: Same as first input
  Sum : Sum  Inputs=|++
  Trigonometric Function : Trigonometry  Operator=cos
  Vector Concatenate : Concatenate  NumInputs=5
  G : Outport
  wires:
  Constant5/1 -> Product5/1
  Trigonometric Function/1 -> Product5/2
  Gain1/1 -> Vector Concatenate/3  "u3"
  Ground/1 -> Vector Concatenate/5, Vector Concatenate/2, Vector Concatenate/1  "u5"
  alpha/1 -> Trigonometric Function/1
  Vector Concatenate/1 -> G/1
  Constant/1 -> Sum/2
  coupled/1 -> Product/1
  Constant4/1 -> Product/2  "u2"
  Sum/1 -> Gain1/1
  Product/1 -> Product5/3, Sum/1
  Product5/1 -> Vector Concatenate/4  "u4"

== system ML_UAV_3D_2/Quadrotor+buoy/6-DOF equations of motion Earth frame/M_1-5 ==
  Rb : Inport
  Rb_T : Inport  Port=2
  alpha,phi : Inport  Port=3
  coupled : Inport  Port=4
  55 : Product
  Constant1 : Constant  Value=m_u*L^2
  Constant2 : Constant  Value=m_u
  Gain1 : Gain  Gain=L
  Ground : Ground
  Ground1 : Ground
  Ground2 : Ground
  Product{,1..2,5..7} (6 alike) : Product
  Signal Specification{1..5} (5 alike) : SignalSpecification  Dimensions=5
  Sum : Sum  Inputs=++|
  Sum1 : Sum  Inputs=++|
  Sum2 : Sum  Inputs=++|
  T, r,xu,xb{1..3,6..7} (5 alike) : Scope
  Vector Concatenate : Concatenate
  Vector Concatenate1 : Concatenate  NumInputs=5  Mode=Multidimensional array  ConcatenateDimension=2
  alpha_ddot : Concatenate  NumInputs=5
  buoy inertia : Subsystem
  c_a : Fcn  Expr=u(3)
  c_a*c_a : Fcn  Expr=u(3)*u(3)
  c_a*c_p : Fcn  Expr=u(3)*u(4)
  c_a*s_p : Fcn  Expr=-u(3)*u(2)
  phi_ddot : Concatenate  NumInputs=5
  s_a*c_p : Fcn  Expr=-u(1)*u(4)
  s_a*s_p : Fcn  Expr=-u(1)*u(2)
  s_alpha s_phi c_alpha c_phi : Trigonometry  Operator=sincos
  x_ddot : Concatenate  NumInputs=5
  y_ddot : Concatenate  NumInputs=5
  z_ddot : Concatenate  NumInputs=5
  M_15 : Outport
  wires:
  Rb/1 -> buoy inertia/1(Rb)
  y_ddot/1 -> Signal Specification2/1
  buoy inertia/1(M11_I) -> Sum/2  "11"
  x_ddot/1 -> Signal Specification1/1, "T, r,xu,xb7"/1
  alpha_ddot/1 -> Signal Specification4/1, "T, r,xu,xb6"/1
  buoy inertia/3(M12_I) -> x_ddot/2, y_ddot/1  "12"
  Product1/1 -> alpha_ddot/1, x_ddot/4, "T, r,xu,xb3"/1  "14"
  buoy inertia/2(M22_I) -> Sum1/2  "22"
  Sum/1 -> x_ddot/1  "11"
  Sum1/1 -> y_ddot/2  "22"
  alpha,phi/1 -> s_alpha s_phi c_alpha c_phi/1
  Constant1/1 -> 55/1, alpha_ddot/4  "44"
  Vector Concatenate1/1 -> M_15/1
  Signal Specification1/1 -> Vector Concatenate1/1
  Signal Specification2/1 -> Vector Concatenate1/2
  Signal Specification3/1 -> Vector Concatenate1/3
  Constant2/1 -> Product/1
  Product2/1 -> alpha_ddot/2, y_ddot/4  "24"
  Product/1 -> "T, r,xu,xb2"/1, Sum1/1, Sum2/1, Sum/1, Gain1/1
  Signal Specification4/1 -> Vector Concatenate1/4
  Signal Specification5/1 -> Vector Concatenate1/5
  z_ddot/1 -> Signal Specification3/1
  Sum2/1 -> z_ddot/3  "33"
  buoy inertia/5(M33_I) -> Sum2/2  "33"
  buoy inertia/4(M13_I) -> z_ddot/1, x_ddot/3  "13"
  buoy inertia/6(M23_I) -> z_ddot/2, y_ddot/3  "23"
  s_alpha s_phi c_alpha c_phi/1 -> Vector Concatenate/1
  s_alpha s_phi c_alpha c_phi/2 -> Vector Concatenate/2
  Vector Concatenate/1 -> c_a*c_p/1, s_a*c_p/1, c_a*s_p/1, s_a*s_p/1, c_a*c_a/1, c_a/1
  s_a*s_p/1 -> Product2/2  "24"
  s_a*c_p/1 -> Product1/2  "14"
  c_a*s_p/1 -> Product6/2  "15"
  c_a*c_p/1 -> Product7/2  "25"
  c_a*c_a/1 -> 55/2  "55"
  c_a/1 -> Product5/2  "34"
  Gain1/1 -> Product5/1, Product7/1, Product2/1, Product6/1, Product1/1
  coupled/1 -> Product/2, "T, r,xu,xb1"/1
  55/1 -> phi_ddot/5  "55"
  Product5/1 -> alpha_ddot/3, z_ddot/4  "43"
  Ground/1 -> z_ddot/5
  Product6/1 -> phi_ddot/1, x_ddot/5  "15"
  Ground1/1 -> alpha_ddot/5
  Product7/1 -> phi_ddot/2, y_ddot/5  "25"
  Ground2/1 -> phi_ddot/4, phi_ddot/3
  phi_ddot/1 -> Signal Specification5/1
  Rb_T/1 -> buoy inertia/2(Rb_T)

== system ML_UAV_3D_2/Quadrotor+buoy/6-DOF equations of motion Earth frame/M_12 ==
  theta : Inport
  Bias : Bias
  Bias1 : Bias
  Signal Specification1 : SignalSpecification  Dimensions=2
  Signal Specification2 : SignalSpecification  Dimensions=2
  Vector Concatenate1 : Concatenate  Mode=Multidimensional array  ConcatenateDimension=2
  Vector Concatenate2 : Concatenate
  Vector Concatenate3 : Concatenate
  added mass : Subsystem
  M_12 : Outport
  wires:
  Signal Specification2/1 -> Vector Concatenate1/2
  Signal Specification1/1 -> Vector Concatenate1/1
  Vector Concatenate1/1 -> M_12/1
  Bias1/1 -> Vector Concatenate3/2
  Bias/1 -> Vector Concatenate2/1
  added mass/2(M22_I) -> Bias1/1
  added mass/3(M12_I) -> Vector Concatenate2/2, Vector Concatenate3/1
  Vector Concatenate2/1 -> Signal Specification1/1
  added mass/1(M11_I) -> Bias/1
  Vector Concatenate3/1 -> Signal Specification2/1
  theta/1 -> added mass/1(theta)

== system ML_UAV_3D_2/Quadrotor+buoy/6-DOF equations of motion Earth frame/Quadrotor Dynamics Outer-Loop ==
  note: Decoupled dynamics
  note: Coupled dynamics
  X15 : Inport
  Xdot15 : Inport  Port=2
  Xddot15 : Inport  Port=3
  coupled : Inport  Port=4
  u1 : Inport  Port=5
  Du : Inport  Port=6
  R_S2C : Inport  Port=7
  R_u_3 : Inport  Port=8
  Add1 : Sum  Inputs=+--
  Constant4 : Constant  Value=m_u
  Data Type Conversion1 : DataTypeConversion  OutDataTypeStr=double
  Delay1 : Delay  DelayLength=1
  Divide : Product  Inputs=*/
  Gu : Subsystem
  IC1 : InitialCondition  Value=pos_u_0_coupled
  IC2 : InitialCondition  Value=[0 0 0]
  IC3 : InitialCondition  Value=pos_u_ini
  IC4 : InitialCondition  Value=v_b_ini
  IC5 : InitialCondition  Value=[pos_b_ini; a_p_0]
  IC6 : InitialCondition  Value=[v_b_ini; 0; 0]
  IC7 : InitialCondition  Value=R_S2C_0
  IC8 : InitialCondition  Value=[pos_b_ini; a_p_0]
  Integrator while decoupled : Subsystem  TreatAsAtomicUnit=on
  Logical Operator : Logic  Operator=NOT  AllPortsSameDT=off
  Mux : Mux  Inputs=2
  Mux1 : Mux  Inputs=2
  Mux2 : Mux  Inputs=2
  Product9 : Product  Inputs=**  SaturateOnIntegerOverflow=on  InputSameDT=on  OutDataTypeStr=Inherit: Same as first input
  Signal Specification1 : SignalSpecification  Dimensions=[3,1]
  Signal Specification2 : SignalSpecification  Dimensions=[3,1]
  Signal Specification7 : SignalSpecification  Dimensions=[3,1]
  Subsystem : Subsystem
  Switch : Switch  Criteria=u2 > Threshold  Threshold=0.5
  Switch1 : Switch  Criteria=u2 > Threshold  Threshold=0.5
  Switch2 : Switch  Criteria=u2 > Threshold  Threshold=0.5
  X1 : InportShadow
  "Xu ddot  " : Scope
  "Xu dot " : Scope
  coupled{1..4} (4 alike) : InportShadow  Port=4
  get initial UAV states for the decoupled dynamics : Subsystem  TreatAsAtomicUnit=on
  is decoupled : Logic  Operator=NOT  AllPortsSameDT=off
  quadrotor position from relative buoy-UAV position : Subsystem
  theta u{1..7} (7 alike) : Scope
  xu init : Scope
  xu1 : Scope
  Xu : Outport
  dot(Xu) : Outport  Port=2
  ddot(Xu) : Outport  Port=3
  wires:
  Subsystem/1(tau_u) -> theta u2/1, Add1/1
  Product9/1 -> Subsystem/1(u1)
  Gu/1(G) -> theta u3/1, Add1/3
  X15/1 -> IC5/1
  Data Type Conversion1/1 -> Product9/1, Gu/1(coupled)
  Add1/1 -> Divide/1
  Logical Operator/1 -> Data Type Conversion1/1
  get initial UAV states for the decoupled dynamics/1(Xu_init) -> xu init/1, IC3/1
  get initial UAV states for the decoupled dynamics/2(Vu_init) -> IC4/1, theta u5/1
  Constant4/1 -> Divide/2
  coupled1/1 -> get initial UAV states for the decoupled dynamics/Trigger
  Du/1 -> Add1/2, theta u4/1
  coupled/1 -> Logical Operator/1
  u1/1 -> Product9/2
  coupled3/1 -> Switch2/2, Switch1/2, Switch/2
  Integrator while decoupled/2("Xu ") -> Mux/2, Switch/3
  quadrotor position from relative buoy-UAV position/1(Xu) -> get initial UAV states for the decoupled dynamics/1(X), IC1/1
  Mux/1 -> xu1/1
  Mux1/1 -> "Xu dot "/1
  Integrator while decoupled/1("dot(Xu) ") -> Mux1/2, Switch1/3
  Mux2/1 -> "Xu ddot  "/1
  Divide/1 -> Mux2/2, Switch2/3, theta u1/1, Integrator while decoupled/1(acc)
  Switch2/1 -> Signal Specification2/1
  Xdot15/1 -> IC6/1
  Xddot15/1 -> quadrotor position from relative buoy-UAV position/3(Xddot15)
  quadrotor position from relative buoy-UAV position/2(Xu_dot) -> get initial UAV states for the decoupled dynamics/2(Xdot), IC2/1
  quadrotor position from relative buoy-UAV position/3(Xu_ddot1) -> Mux2/1, Switch2/1
  is decoupled/1 -> theta u6/1, Integrator while decoupled/Enable
  coupled2/1 -> Delay1/1, is decoupled/1, theta u7/1
  Switch1/1 -> Signal Specification1/1
  coupled4/1 -> quadrotor position from relative buoy-UAV position/Enable
  Switch/1 -> Signal Specification7/1
  [Vu_init] -> Integrator while decoupled/2(X dot init)
  [Xu_init] -> Integrator while decoupled/3(X init)
  X1/1 -> IC8/1
  Delay1/1 -> Integrator while decoupled/5(reset)
  IC3/1 -> [Xu_init]
  IC4/1 -> [Vu_init]
  IC1/1 -> Mux/1, Switch/1
  IC2/1 -> Switch1/1, Mux1/1
  IC5/1 -> quadrotor position from relative buoy-UAV position/1(X15)
  IC8/1 -> Integrator while decoupled/4(X123)
  IC6/1 -> quadrotor position from relative buoy-UAV position/2(Xdot15)
  R_S2C/1 -> IC7/1
  IC7/1 -> quadrotor position from relative buoy-UAV position/4(R_S2C)
  R_u_3/1 -> Subsystem/2(R_u_3)
  Signal Specification7/1 -> Xu/1
  Signal Specification1/1 -> dot(Xu)/1
  Signal Specification2/1 -> ddot(Xu)/1

== system ML_UAV_3D_2/Quadrotor+buoy/6-DOF equations of motion Earth frame/Rigid Body Torque Equations  ==
  note: 1-phi: roll
      | 2-theta: pitch
      | 3-psi: yaw
  M_body : Inport
  I : Inport  Port=2
  Reset : Inport  Port=3
  " Euler" : DiscreteIntegrator  ExternalReset=sampled level  InitialCondition=euler0  SampleTime=-1  ICPrevOutput=DiscIntNeverNeededParam  ICPrevScaledInput=DiscIntNeverNeededParam
  " omega" : DiscreteIntegrator  ExternalReset=sampled level  InitialCondition=omega0  SampleTime=-1  ICPrevOutput=DiscIntNeverNeededParam  ICPrevScaledInput=DiscIntNeverNeededParam
  Constant : Constant  Value=[0 0 0]
  Euler : Integrator  Commented=on  ExternalReset=level hold  InitialCondition=[Phi0 Theta0 Psi0]  UpperSaturationLimit=2  LowerSaturationLimit=-2
  I.w : Product  Multiplication=Matrix(*)
  I.w_dot : Sum  Inputs=-+
  Product : Product  Multiplication=Matrix(*)
  "Reset " : InportShadow  Port=3
  "Reset  " : InportShadow  Port=3
  Rotation Angles to Angular transformation matrix body to earth Rotation Order: ZXY : Subsystem  AncestorBlock=|  mask(Ang2T){}
      | UAV_Control/Rotation Angles to
      | Angular transformation matrix
      | body to earth
      | Rotation Order: ZXY
      mask help: Determine the 3-by-3 Angular transformation matrix (T) from a given set of rotation angles (ZXY).
      mask Help:
      | Generate the Angular Transformation matrix (T) from the Euler angles. Order of transformation. body to earth.
      | ZYX
      | 
      | T_B2E = [         cos(theta)             0          -sin(theta)
      |                  -sin(theta)*tan(phi)      1    -cos(theta)*tan(phi)
      |                    sin(theta)/cos(phi)     0     cos(theta)/cos(phi) ]
      mask Display:
      | port_label('input',1,'[R_1,R_2,R_3]','texmode','on')
      | port_label('output',1,'T_{eb}','texmode','on')
  Rotation Angles to Direction Cosine Matrix body to earth Rotation Order: ZXY : UAV_Control/Rotation Angles to Direction Cosine Matrix body to earth Rotation Order: ZXY
      settings: SourceProductName=UAV_Control
  Switch : Switch  Criteria=u2 > Threshold  Threshold=0.5
  "omega  " : Integrator  Commented=on  ExternalReset=level hold  InitialCondition=omega0  UpperSaturationLimit=2  LowerSaturationLimit=-2
  w x (I.w) : UAV_Control/3x3 Cross Product
      settings: SourceProductName=UAV_Control
  w_dot : Product  Inputs=/*  Multiplication=Matrix(*)
  "Euler " : Outport
  omega : Outport  Port=2
  omega_dot : Outport  Port=3
  DCM_b2e : Outport  Port=4
  wires:
  w x (I.w)/1 -> I.w_dot/1
  M_body/1 -> I.w_dot/2
  " Euler"/1 -> "Euler "/1, Rotation Angles to Direction Cosine Matrix body to earth Rotation Order: ZXY/1, Rotation Angles to Angular transformation matrix body to earth Rotation Order: ZXY/1(R1,R2,R3)
  Rotation Angles to Angular transformation matrix body to earth Rotation Order: ZXY/1(T) -> Product/1
  w_dot/1 -> " omega"/1, Switch/3
  Product/1 -> " Euler"/1
  I/1 -> I.w/1, w_dot/1
  " omega"/1 -> Product/2, I.w/2, w x (I.w)/1, omega/1
  Constant/1 -> Switch/1
  Reset/1 -> Switch/2
  Switch/1 -> omega_dot/1
  "Reset "/1 -> " omega"/2
  "Reset  "/1 -> " Euler"/2
  Rotation Angles to Direction Cosine Matrix body to earth Rotation Order: ZXY/1 -> DCM_b2e/1
  I.w/1 -> w x (I.w)/2
  I.w_dot/1 -> w_dot/2

== system ML_UAV_3D_2/Quadrotor+buoy/6-DOF equations of motion Earth frame/Tension from Buoy, X direction ==
  alpha : Inport
  M12 : Inport  Port=2
  D12 : Inport  Port=3
  Vr,Wr : Inport  Port=4
  Xb_ddot : Inport  Port=5
  G : Inport  Port=6
  FB : Inport  Port=7
  Add1 : Sum  Inputs=+++-
  Constant : Constant  Value=0
  Math Function : Math  Operator=reciprocal  SaturateOnIntegerOverflow=on
  Math Function1 : Math  Operator=reciprocal  SaturateOnIntegerOverflow=on
  Product1 : Product
  Product2 : Product  Inputs=**  Multiplication=Matrix(*)
  Product3 : Product  Inputs=**  Multiplication=Matrix(*)
  Scope5 : Scope
  Trigonometric Function3 : Trigonometry  Operator=sincos
  Vector Concatenate2 : Concatenate
  Vector Concatenate3 : Concatenate
  T x,z : Outport
  wires:
  alpha/1 -> Trigonometric Function3/1
  M12/1 -> Product2/1
  Vr,Wr/1 -> Product3/2
  D12/1 -> Product3/1
  Xb_ddot/1 -> Product2/2
  G/1 -> Add1/3
  Product2/1 -> Add1/2
  Trigonometric Function3/2 -> Math Function/1
  Trigonometric Function3/1 -> Math Function1/1
  Product3/1 -> Add1/1
  Math Function/1 -> Vector Concatenate2/1
  Math Function1/1 -> Vector Concatenate2/2
  Constant/1 -> Vector Concatenate3/1
  Vector Concatenate3/1 -> Add1/4
  FB/1 -> Vector Concatenate3/2
  Product1/1 -> Scope5/1, T x,z/1
  Vector Concatenate2/1 -> Product1/2
  Add1/1 -> Product1/1

== system ML_UAV_3D_2/Quadrotor+buoy/6-DOF equations of motion Earth frame/Tension from UAV, X and r directions ==
  note: something wrong, there should be ne r_ddot, but alpha dot and phidot
  note: ?? eq 33, ur?
  alpha : Inport
  r_p_ddot : Inport  Port=2
  euler_u : Inport  Port=3
  u1 : Inport  Port=4
  Xb_ddot : Inport  Port=5
  Xu_ddot : Inport  Port=6
  R_C2S : Inport  Port=7
  "R_b2e_u " : Inport  Port=8
  coupled : Inport  Port=9
  1 3 : Selector  Commented=on  NumberOfDimensions=2  InputPortWidth=3  IndexOptions=Index vector (dialog),Index vector (dialog)  Indices=[1],[3]  OutputSizes=1,1
  Add1 : Sum  Commented=on  Inputs=+-+
  Add2 : Sum  Commented=on  Inputs=---
  Add3 : Sum  Commented=on  Inputs=+-
  Discrete Derivative2 : simulink/Discrete/Discrete Derivative  Commented=on  gainval=1.0  ICPrevScaledInput=L*500  OutMin=[]  OutMax=[]  OutDataType=fixdt(1, 16)  OutScaling=2^-10  DoSatur=off
  Discrete Derivative3 : simulink/Discrete/Discrete Derivative  Commented=on  gainval=1.0  ICPrevScaledInput=0  OutMin=[]  OutMax=[]  OutDataType=fixdt(1, 16)  OutScaling=2^-10  DoSatur=off
  Gain14 : Gain  Commented=on
  Gain15 : Gain  Commented=on  Gain=m_u
  Gain5 : Gain  Commented=on  Gain=m_u
  Gain6 : Gain  Commented=on  Gain=m_u*g
  Product1 : Product  Commented=on  Multiplication=Matrix(*)
  Product10 : Product  Commented=on  Inputs=**  Multiplication=Matrix(*)
  Product12 : Product  Commented=on
  Product2 : Product  Commented=on
  Product9 : Product  Commented=on  Inputs=*/
  R_C2S1 : InportShadow  Port=7
  Selector1 : Selector  Commented=on  NumberOfDimensions=2  InputPortWidth=3  IndexOptions=Index vector (dialog),Index vector (dialog)  Indices=[1],[1 2 3]  OutputSizes=1,1
  Signal Specification1 : SignalSpecification  Commented=on  Dimensions=1
  Signal Specification5 : SignalSpecification  Commented=on  Dimensions=1
  Signal Specification6 : SignalSpecification  Commented=on  Dimensions=1
  "T, r,xu,xb1" : Scope  Commented=on
  "T, r,xu,xb2" : Scope  Commented=on
  "T, r,xu,xb3" : Scope  Commented=on
  "Tension from UAV, z direction" : Subsystem
  Trigonometric Function3 : Trigonometry  Commented=on
  Trigonometric Function6 : Trigonometry  Commented=on  Operator=cos
  Trigonometric Function8 : Trigonometry  Commented=on
  Xu_ddot1 : InportShadow  Port=6
  alpha1 : InportShadow
  r : Constant  Commented=on  Value=L
  "u1 " : InportShadow  Port=4
  x_ddot1 : Selector  Commented=on  InputPortWidth=2  IndexOptions=Index vector (dialog)  Indices=1  OutputSizes=1
  "T, from r" : Outport
  "T, from uav z" : Outport  Port=2
  wires:
  r/1 -> Discrete Derivative2/1
  r_p_ddot/1 -> Add2/1
  alpha/1 -> Trigonometric Function3/1
  Add2/1 -> Gain5/1
  Discrete Derivative2/1 -> Discrete Derivative3/1
  Trigonometric Function3/1 -> Signal Specification5/1
  Gain5/1 -> "T, r,xu,xb1"/1, Add1/1
  Gain6/1 -> "T, r,xu,xb2"/1, Add1/2
  Add3/1 -> Product9/1
  Gain14/1 -> Add3/1
  Trigonometric Function8/1 -> Product12/1
  "u1 "/1 -> "Tension from UAV, z direction"/3(u1), Product12/2
  alpha1/1 -> "Tension from UAV, z direction"/1(alpha), Trigonometric Function6/1
  Product12/1 -> Gain14/1
  x_ddot1/1 -> Gain15/1
  Trigonometric Function6/1 -> Product9/2
  Xu_ddot/1 -> x_ddot1/1
  euler_u/1 -> "Tension from UAV, z direction"/2(euler_u), Trigonometric Function8/1
  Gain15/1 -> Add3/2
  Product2/1 -> Signal Specification6/1
  Xb_ddot/1 -> Product10/2
  Add1/1 -> Signal Specification1/1
  Discrete Derivative3/1 -> Add2/3
  Signal Specification5/1 -> Gain6/1
  Signal Specification6/1 -> "T, r,xu,xb3"/1, Add1/3
  Signal Specification1/1 -> "T, from r"/1
  Xu_ddot1/1 -> "Tension from UAV, z direction"/4(Xu_ddot)
  R_C2S/1 -> Selector1/1
  "R_b2e_u "/1 -> Product1/1
  R_C2S1/1 -> Product1/2
  Product1/1 -> 1 3/1
  u1/1 -> Product2/2
  1 3/1 -> Product2/1
  Product10/1 -> Add2/2
  Selector1/1 -> Product10/1
  coupled/1 -> "Tension from UAV, z direction"/Enable
  "Tension from UAV, z direction"/1("T, from z simple") -> "T, from uav z"/1
